simulink model "fun"  (R2022b)
settings: Solver=VariableStepAuto  StartTime=0.0  StopTime=10.0  RelTol=1e-3
undefined symbols (not defined in the file): fy3tab, h, k1, k2, m1, m2, m3, x0, xp0, y2p0, y30, y3p0, y3tab
libraries: simulink x1
settings Model: Creator=morde  LastModifiedBy=morde

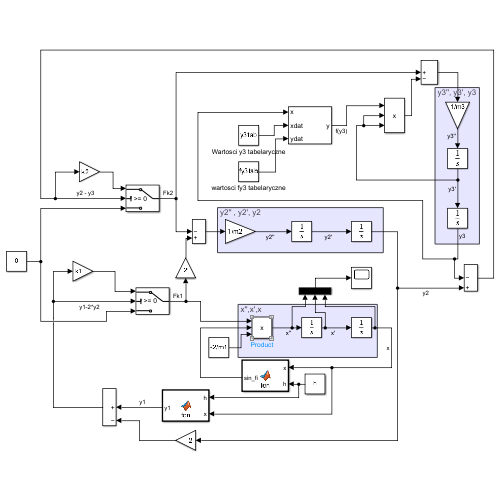
[thumbnail: Simulink's stored preview of the top-level diagram]
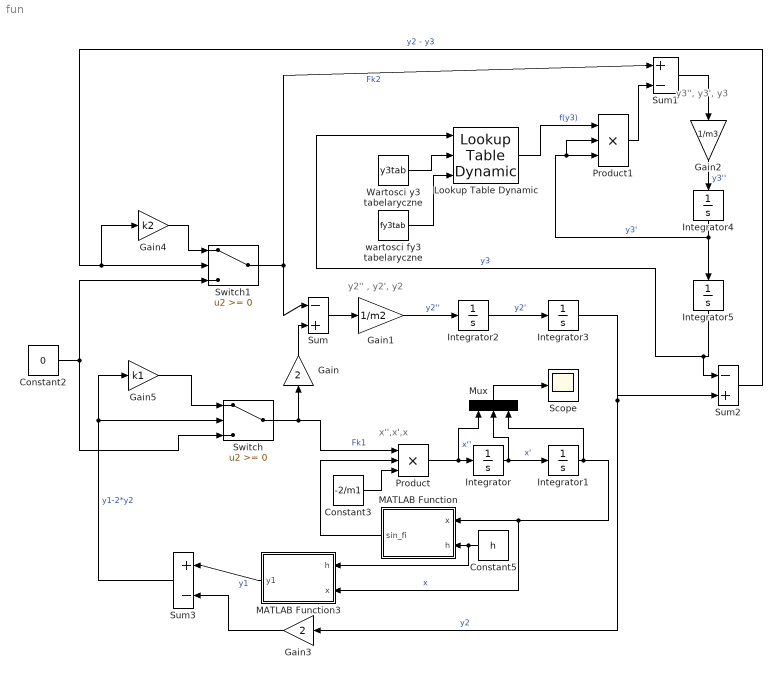
== system fun ==
  note: x'',x',x
  note: y3'', y3', y3
  note: y2'' , y2', y2
  Constant2 : Constant  Value=0
  Constant3 : Constant  Value=-2/m1
  Constant5 : Constant  Value=h
  Gain : Gain  Gain=2
  Gain1 : Gain  Gain=1/m2
  Gain2 : Gain  Gain=1/m3
  Gain3 : Gain  Gain=2
  Gain4 : Gain  Gain=k2
  Gain5 : Gain  Gain=k1
  Integrator : Integrator  InitialCondition=xp0
  Integrator1 : Integrator  InitialCondition=x0
  Integrator2 : Integrator  InitialCondition=y2p0
  Integrator3 : Integrator
  Integrator4 : Integrator  InitialCondition=y3p0
  Integrator5 : Integrator  InitialCondition=y30
  Lookup Table Dynamic : simulink/Lookup Tables/Lookup Table Dynamic  LookUpMeth=Interpolation-Use End Values  OutDataType=fixdt('double')  OutScaling=[]  OutputDataTypeScalingMode=Specify via dialog  OutDataTypeStr=double  DoSatur=off
  MATLAB Function : MATLAB Function  TreatAsAtomicUnit=on
  MATLAB Function3 : MATLAB Function  TreatAsAtomicUnit=on
  Mux : Mux  Inputs=3
  Product : Product  Inputs=3
  Product1 : Product  Inputs=3
  Scope : Scope
  Sum : Sum  Inputs=|-+
  Sum1 : Sum  Inputs=|+-
  Sum2 : Sum  Inputs=|-+
  Sum3 : Sum  Inputs=|+-
  Switch : Switch  SaturateOnIntegerOverflow=off  InputSameDT=off
  Switch1 : Switch  SaturateOnIntegerOverflow=off  InputSameDT=off
  Wartosci y3 tabelaryczne : Constant  Value=y3tab
  wartosci fy3 tabelaryczne : Constant  Value=fy3tab
  wires:
  Wartosci y3 tabelaryczne/1 -> Lookup Table Dynamic/2
  wartosci fy3 tabelaryczne/1 -> Lookup Table Dynamic/3
  Sum3/1 -> Switch/2, Gain5/1  "y1-2*y2"
  Product/1 -> Mux/1, Integrator/1  "x''"
  Switch/1 -> Product/1, Gain/1  "Fk1"
  MATLAB Function/1(sin_fi) -> Product/2
  Constant3/1 -> Product/3
  Integrator/1 -> Mux/2, Integrator1/1  "x'"
  Integrator1/1 -> Mux/3, MATLAB Function3/2(x), MATLAB Function/1(x)  "x"
  Constant5/1 -> MATLAB Function3/1(h), MATLAB Function/2(h)
  Sum2/1 -> Gain4/1, Switch1/2  "y2 - y3"
  Constant2/1 -> Switch/3, Switch1/3
  Switch1/1 -> Sum1/1, Sum/1  "Fk2"
  Gain/1 -> Sum/2
  Sum/1 -> Gain1/1
  Gain1/1 -> Integrator2/1  "y2''"
  Integrator2/1 -> Integrator3/1  "y2'"
  Integrator5/1 -> Sum2/1, Lookup Table Dynamic/1  "y3"
  Lookup Table Dynamic/1 -> Product1/1  "f(y3)"
  Sum1/1 -> Gain2/1
  Gain2/1 -> Integrator4/1  "y3''"
  Integrator4/1 -> Product1/3, Product1/2, Integrator5/1  "y3'"
  Integrator3/1 -> Gain3/1, Sum2/2  "y2"
  MATLAB Function3/1(y1) -> Sum3/1  "y1"
  Gain3/1 -> Sum3/2
  Mux/1 -> Scope/1
  Gain4/1 -> Switch1/1
  Gain5/1 -> Switch/1
  Product1/1 -> Sum1/2

== matlab function fun/MATLAB Function3 ==
  data: h input; x input; y1 output
function y1 = fcn(h, x)

y1 = sqrt(x^2 + h^2) - h;

== matlab function fun/MATLAB Function ==
  data: x input; sin_fi output; h input

function sin_fi = fcn(x,h)

sin_fi = x/sqrt(x^2+h^2);
